simulink library "rayTrace_ul"  (R2018b)
settings: Solver=VariableStepAuto  StartTime=0.0  StopTime=10.0  RelTol=1e-3
values from neighbouring files (symbols this model uses):
  grnd2CamRotMat = calculateRotationMatrix(roll,pitch,yaw)    [rayTrace_ts.m]    (also in rayTrace_ts1.m = calculateRotationMatrix(roll_rad,pitch,yaw_rad); rayTrace_ts2.m; snellDotPosition_init.m = calculateRotationMatrix(     cameraEulerAngles_rad(1),     c; snellDotPosition_ts.m)
settings Model: Creator=MAE-NCSUCORE  LastModifiedBy=mcobb

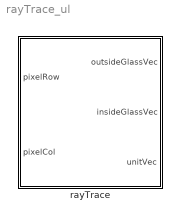
== system rayTrace_ul ==
  rayTrace : Subsystem  mask{camPosVec_cm=[1 1 1], camEulAngles_deg=[0 0 0], dist2Glass_cm=0, indOfRefVec=[0 0 0], glassPlane=0, glassThickness_cm=0, imageDimsVec_px=[1000 2000], camFOV_deg=0}
      mask prompts: camPosVec_cm "Camera Position Vector, cm"; camEulAngles_deg "Camera Euler Angles, deg"; dist2Glass_cm "Distance to glass, cm"; indOfRefVec "Indices of refraction [air glass water]"; glassPlane "Glass plane (1 = xy, 2 = xz)"; glassThickness_cm "Glass thickness, cm"; imageDimsVec_px "Image dimensions, px [rows cols]"; camFOV_deg "Camera field of view angles,deg  [horiz vert]"
      mask init:
      | rayTrace_init

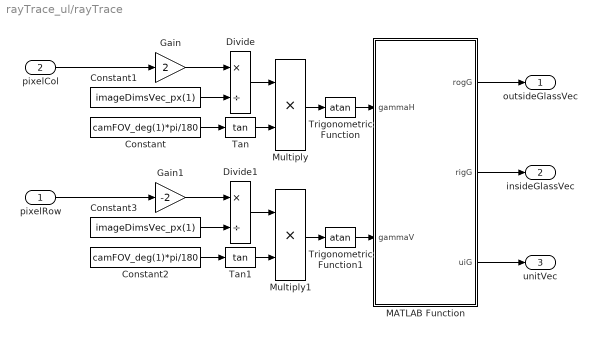
== system rayTrace_ul/rayTrace ==
  pixelRow : Inport
  pixelCol : Inport  Port=2
  Constant : Constant  Value=camFOV_deg(1)*pi/180
  Constant1 : Constant  Value=imageDimsVec_px(1)
  Constant2 : Constant  Value=camFOV_deg(1)*pi/180
  Constant3 : Constant  Value=imageDimsVec_px(1)
  Divide : Product  Inputs=*/
  Divide1 : Product  Inputs=*/
  Gain : Gain  Gain=2
  Gain1 : Gain  Gain=-2
  MATLAB Function : MATLAB Function  TreatAsAtomicUnit=on
  Multiply : Product
  Multiply1 : Product
  Tan : Trigonometry  Operator=tan
  Tan1 : Trigonometry  Operator=tan
  Trigonometric Function : Trigonometry  Operator=atan
  Trigonometric Function1 : Trigonometry  Operator=atan
  outsideGlassVec : Outport
  insideGlassVec : Outport  Port=2
  unitVec : Outport  Port=3
  wires:
  MATLAB Function/2(rigG) -> insideGlassVec/1
  MATLAB Function/3(uiG) -> unitVec/1
  MATLAB Function/1(rogG) -> outsideGlassVec/1
  Trigonometric Function/1 -> MATLAB Function/1(gammaH)
  Multiply/1 -> Trigonometric Function/1
  Tan/1 -> Multiply/2
  Constant/1 -> Tan/1
  Divide/1 -> Multiply/1
  Gain/1 -> Divide/1
  Constant1/1 -> Divide/2
  Gain1/1 -> Divide1/1
  Constant3/1 -> Divide1/2
  Constant2/1 -> Tan1/1
  Trigonometric Function1/1 -> MATLAB Function/2(gammaV)
  Multiply1/1 -> Trigonometric Function1/1
  Tan1/1 -> Multiply1/2
  Divide1/1 -> Multiply1/1
  pixelRow/1 -> Gain1/1
  pixelCol/1 -> Gain/1

== matlab function rayTrace_ul/rayTrace/MATLAB Function ==
  data: rogG output; gammaH input; gammaV input; rigG output; uiG output; camPosVec_cm parameter; grnd2CamRotMat parameter; dist2Glass_cm parameter; indOfRefVec parameter; glassPlane parameter; glassThickness_cm parameter
function [rogG,rigG,uiG] = ...
    rayTrace(gammaH,gammaV,camPosVec_cm, grnd2CamRotMat, dist2Glass_cm, indOfRefVec,...
glassPlane, glassThickness_cm)

[rogG,rigG,uiG] = ...
    rayTrace(camPosVec_cm,grnd2CamRotMat,dist2Glass_cm,gammaH,gammaV,...
    indOfRefVec,glassPlane,glassThickness_cm);
